simulink model "simulink_model"  (R2024b)
settings: Solver=ode45  StartTime=0.0  StopTime=2.0  RelTol=1e-5

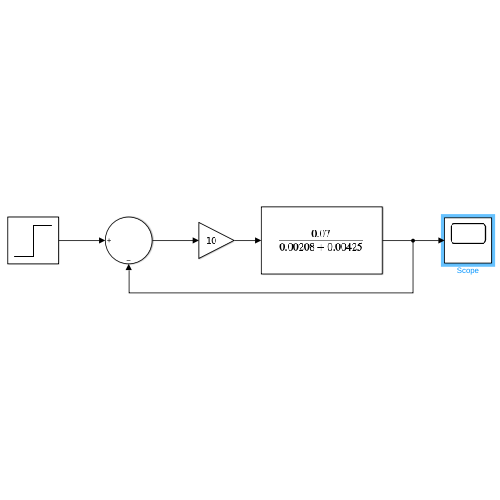
[thumbnail: Simulink's stored preview of the top-level diagram]
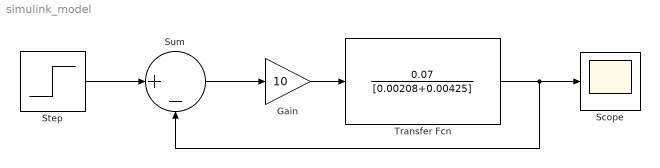
== system simulink_model ==
  Gain : Gain  Gain=10
  Scope : Scope
  Step : Step  Time=0  SampleTime=0
  Sum : Sum  Inputs=|+-
  Transfer Fcn : TransferFcn  Numerator=[0.07]  Denominator=[0.00208+0.00425]
  wires:
  Sum/1 -> Gain/1
  Gain/1 -> Transfer Fcn/1
  Step/1 -> Sum/1
  Transfer Fcn/1 -> Sum/2, Scope/1
